simulink model "CH23_2C1"  (R2021b)
settings: Solver=ode45  StartTime=0.0  StopTime=50  RelTol=1e-3  EnableMultiTasking=on
libraries: commrandsrc2 x1, commdigbbndam3 x1
settings Model: Creator=my2  LastModifiedBy=IT
settings SolverCC: AlgebraicLoopSolver=TrustRegion
settings DataIOCC: LimitDataPoints=on  SaveFormat=Array  SignalLoggingSaveFormat=ModelDataLogs  ReturnWorkspaceOutputs=off
settings OptimizationCC: LifeSpan=inf
settings DebuggingCC: SolverPrmCheckMsg=warning  MultiTaskDSMMsg=warning  MultiTaskCondExecSysMsg=none  FcnCallInpInsideContextMsg=warning  SFUnexpectedBacktrackingDiag=warning  SFNoUnconditionalDefaultTransitionDiag=warning  SFExecutionAtInitializationDiag=none  SFMachineParentedDataDiag=warning  ArithmeticOperatorsInVariantConditions=warning
settings HardwareCC: ProdBitPerPointer=32  ProdBitPerSizeT=32  ProdBitPerPtrDiffT=32  ProdLargestAtomicFloat=None  ProdIntDivRoundTo=Undefined  ProdEndianess=Unspecified  ProdWordSize=32  ProdHWDeviceType=32-bit Generic
settings ModelReferenceCC: PropagateSignalLabelsOutOfModel=off
settings SFSimCC: SimUseLocalCustomCode=off  CustomCodeUndefinedFunction=UseInterfaceOnly
settings RTWCC: RTWUseLocalCustomCode=off
settings CodeAppCC: StateflowObjectComments=on
settings GRTTargetCC: TargetLangStandard=C89/C90 (ANSI)  CombineOutputUpdateFcns=off  GRTInterface=on
settings ConfigComp: CovMetricSettings=dw  CovSaveCumulativeToWorkspaceVar=on  CovSaveSingleToWorkspaceVar=on  CovExternalEMLEnable=off

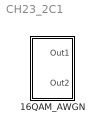
== system CH23_2C1 ==
  16QAM_AWGN : Subsystem

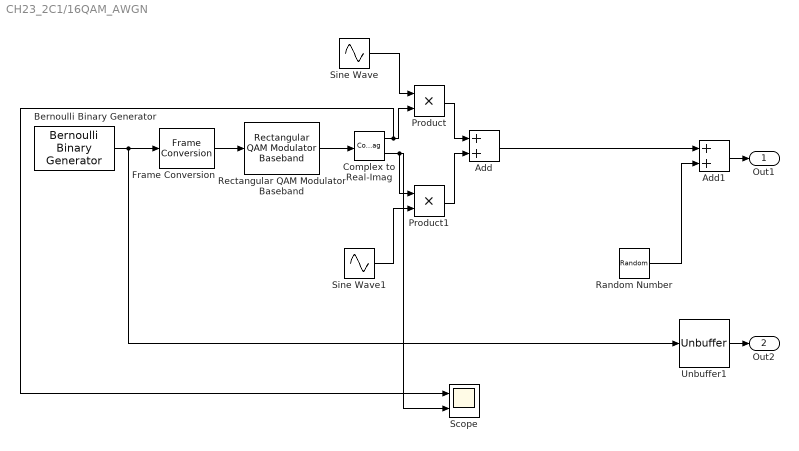
== system CH23_2C1/16QAM_AWGN ==
  Add : Sum
  Add1 : Sum
  Bernoulli Binary Generator : commrandsrc2/Bernoulli Binary Generator  P=0.5  seed=20301181  Ts=1  frameBased=on  sampPerFrame=4  orient=off  outDataType=boolean
      settings: SourceProductBaseCode=CM
  Complex to Real-Imag : ComplexToRealImag
  Frame Conversion : FrameConversion  OutFrame=Sample-based
  Product : Product
  Product1 : Product
  Random Number : RandomNumber  Variance=0  Seed=41  SampleTime=1/100  VectorParams1D=off
  Rectangular QAM Modulator Baseband : commdigbbndam3/Rectangular QAM Modulator Baseband  M=16  InType=Bit  Enc=Gray  Mapping=[0:15]  PowType=Min. distance between symbols  MinDist=2  AvgPow=1  PeakPow=1  Ph=0  outDtype=double  outWordLen=16  outUDDataType=sfix(16)  outFracLenMode=Best precision  outFracLen=15  outDataTypeStr=double  outLastDataTypeStr=double
  Scope : Scope  NumInputPorts=2
  Sine Wave : Sin  SampleTime=1/100
  Sine Wave1 : Sin  SampleTime=1/100
  Unbuffer1 : Unbuffer
  Out1 : Outport
  Out2 : Outport  Port=2
  wires:
  Complex to Real-Imag/2 -> Scope/2, Product1/1
  Unbuffer1/1 -> Out2/1
  Add1/1 -> Out1/1
  Random Number/1 -> Add1/2
  Complex to Real-Imag/1 -> Scope/1, Product/2
  Sine Wave/1 -> Product/1
  Rectangular QAM Modulator Baseband/1 -> Complex to Real-Imag/1
  Frame Conversion/1 -> Rectangular QAM Modulator Baseband/1
  Bernoulli Binary Generator/1 -> Frame Conversion/1, Unbuffer1/1
  Product/1 -> Add/1
  Sine Wave1/1 -> Product1/2
  Add/1 -> Add1/1
  Product1/1 -> Add/2
